simulink model "SF053A_HwAgVehCentrTrim"  (R2013b)
settings: Solver=FixedStepDiscrete  SolverMode=SingleTasking  StartTime=0.0  StopTime=1  FixedStep=0.002  RelTol=1e-3
values from neighbouring files (symbols this model uses):
  ENGRUNACTVTRUE_CNT_U08 = DataDict.Constant    [SF053A_HwAgVehCentrTrim_DataDict.m]
  HWAGCLRTRIMPRFMD_CNT_LGC = DataDict.Constant    [SF053A_HwAgVehCentrTrim_DataDict.m]
  HWAGCLRVAL_HWDEG_F32 = DataDict.Constant    [SF053A_HwAgVehCentrTrim_DataDict.m]
  HWAGEOTCCWNOTDETD_CNT_U08 = DataDict.Constant    [SF053A_HwAgVehCentrTrim_DataDict.m]
  HWAGEOTCWNOTDETD_CNT_U08 = DataDict.Constant    [SF053A_HwAgVehCentrTrim_DataDict.m]
  HWAGMAGTHDEXCDD_CNT_U08 = DataDict.Constant    [SF053A_HwAgVehCentrTrim_DataDict.m]
  HWAGTRIMPRFMD_CNT_LGC = DataDict.Constant    [SF053A_HwAgVehCentrTrim_DataDict.m]
  HwAgVehCentrTrimHwAgLim = DataDict.Calibration    [SF053A_HwAgVehCentrTrim_DataDict.m]
  HwAgVehCentrTrimVehSpdMaxThd = DataDict.Calibration    [SF053A_HwAgVehCentrTrim_DataDict.m]
  HwAgVehCentrTrimVld = DataDict.NTC    [SF053A_HwAgVehCentrTrim_DataDict.m]
  NODEBSTEP_CNT_U16 = DataDict.Constant    [SF053A_HwAgVehCentrTrim_DataDict.m]
  UPDHWAGTRIMPRFMD_CNT_U08 = DataDict.Constant    [SF053A_HwAgVehCentrTrim_DataDict.m]
  VEHSPDTHDEXCDD_CNT_U08 = DataDict.Constant    [SF053A_HwAgVehCentrTrim_DataDict.m]
undefined symbols (not defined in the file or in its folder): NtcSts1, u2, u3, u4, u5
libraries: simulink x6, NxtrNvM x3, NxtrLim x2
(part 2 of 3)

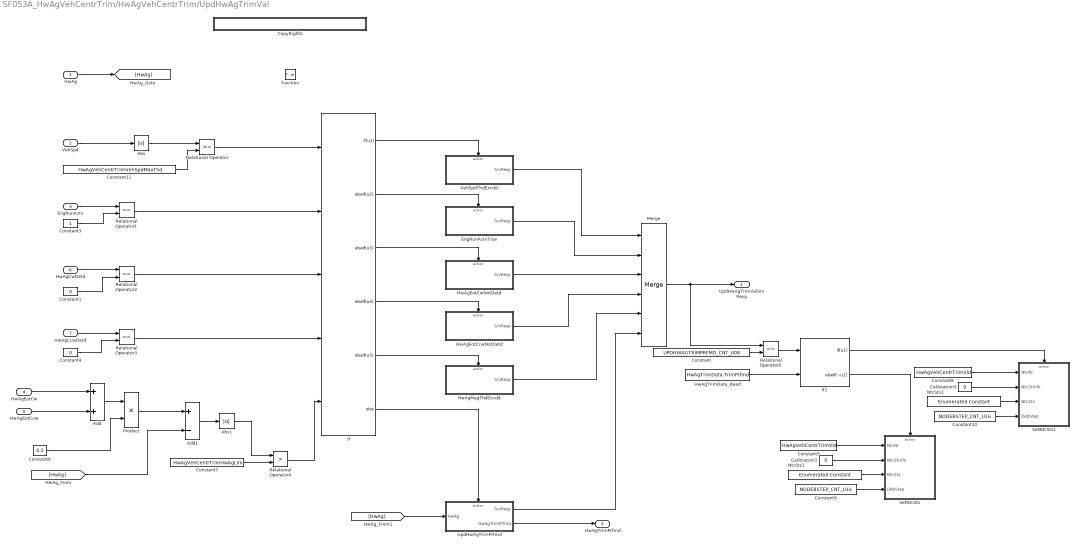
== system SF053A_HwAgVehCentrTrim/HwAgVehCentrTrim/UpdHwAgTrimVal ==
  HwAg : Inport
  VehSpd : Inport  RequirementInfo="{'linktype_rmi_doors' '0000babb (/E-STEER Core/SubSystem Specifications/Application Functions/SF053A Handwheel Angle Vehicle Center Trim)' '#SF053A_32' 'true' 'REQ:  SF053A_32' '' ; 'linktype_rmi_doors' '0000babb (/E-STEER Core/SubSystem Specifications/Application Functions/SF053A Handwheel Angle Vehicle Center Trim)' '#SF053A_79' 'true' 'REQ:  SF053A_79' '' } %GIDa_a63d72e2_7325_4356_9d1e_f8480a82d0d4"  Port=2
  EngRunActv : Inport  RequirementInfo="{'linktype_rmi_doors' '0000babb (/E-STEER Core/SubSystem Specifications/Application Functions/SF053A Handwheel Angle Vehicle Center Trim)' '#SF053A_32' 'true' 'REQ:  SF053A_32' '' ; 'linktype_rmi_doors' '0000babb (/E-STEER Core/SubSystem Specifications/Application Functions/SF053A Handwheel Angle Vehicle Center Trim)' '#SF053A_79' 'true' 'REQ:  SF053A_79' '' } %GIDa_7bfd1cfe_a81d_4c20_a64c_d0273af8ffe3"  Port=3
  HwAgEotCw : Inport  RequirementInfo="{'linktype_rmi_doors' '0000babb (/E-STEER Core/SubSystem Specifications/Application Functions/SF053A Handwheel Angle Vehicle Center Trim)' '#SF053A_32' 'true' 'REQ:  SF053A_32' '' ; 'linktype_rmi_doors' '0000babb (/E-STEER Core/SubSystem Specifications/Application Functions/SF053A Handwheel Angle Vehicle Center Trim)' '#SF053A_79' 'true' 'REQ:  SF053A_79' '' } %GIDa_18a440d3_64a6_4375_b85b_cbfdb945b10b"  Port=4
  HwAgEotCcw : Inport  RequirementInfo="{'linktype_rmi_doors' '0000babb (/E-STEER Core/SubSystem Specifications/Application Functions/SF053A Handwheel Angle Vehicle Center Trim)' '#SF053A_32' 'true' 'REQ:  SF053A_32' '' ; 'linktype_rmi_doors' '0000babb (/E-STEER Core/SubSystem Specifications/Application Functions/SF053A Handwheel Angle Vehicle Center Trim)' '#SF053A_79' 'true' 'REQ:  SF053A_79' '' } %GIDa_1e2d1dde_4459_46e8_93f9_57f17d4f6490"  Port=5
  HwAgCwDetd : Inport  RequirementInfo="{'linktype_rmi_doors' '0000babb (/E-STEER Core/SubSystem Specifications/Application Functions/SF053A Handwheel Angle Vehicle Center Trim)' '#SF053A_32' 'true' 'REQ:  SF053A_32' '' ; 'linktype_rmi_doors' '0000babb (/E-STEER Core/SubSystem Specifications/Application Functions/SF053A Handwheel Angle Vehicle Center Trim)' '#SF053A_79' 'true' 'REQ:  SF053A_79' '' } %GIDa_ce18ba93_be2d_4182_b1c9_fe28610a3b2f"  Port=6
  HwAgCcwDetd : Inport  RequirementInfo="{'linktype_rmi_doors' '0000babb (/E-STEER Core/SubSystem Specifications/Application Functions/SF053A Handwheel Angle Vehicle Center Trim)' '#SF053A_32' 'true' 'REQ:  SF053A_32' '' ; 'linktype_rmi_doors' '0000babb (/E-STEER Core/SubSystem Specifications/Application Functions/SF053A Handwheel Angle Vehicle Center Trim)' '#SF053A_79' 'true' 'REQ:  SF053A_79' '' } %GIDa_ef525b95_af54_48f7_86e9_a1604fe43558"  Port=7
  function : TriggerPort  TriggerType=function-call
  Abs : Abs  RequirementInfo="{'linktype_rmi_doors' '0000babb (/E-STEER Core/SubSystem Specifications/Application Functions/SF053A Handwheel Angle Vehicle Center Trim)' '#SF053A_32' 'true' 'REQ:  SF053A_32' '' ; 'linktype_rmi_doors' '0000babb (/E-STEER Core/SubSystem Specifications/Application Functions/SF053A Handwheel Angle Vehicle Center Trim)' '#SF053A_79' 'true' 'REQ:  SF053A_79' '' } %GIDa_d991774f_80ee_4fb7_a63e_280bffb35c40"
  Abs1 : Abs  RequirementInfo="{'linktype_rmi_doors' '0000babb (/E-STEER Core/SubSystem Specifications/Application Functions/SF053A Handwheel Angle Vehicle Center Trim)' '#SF053A_32' 'true' 'REQ:  SF053A_32' '' ; 'linktype_rmi_doors' '0000babb (/E-STEER Core/SubSystem Specifications/Application Functions/SF053A Handwheel Angle Vehicle Center Trim)' '#SF053A_79' 'true' 'REQ:  SF053A_79' '' } %GIDa_67f6e9b9_3d0b_4591_be2f_c526e2159446"
  Add : Sum  RequirementInfo="{'linktype_rmi_doors' '0000babb (/E-STEER Core/SubSystem Specifications/Application Functions/SF053A Handwheel Angle Vehicle Center Trim)' '#SF053A_32' 'true' 'REQ:  SF053A_32' '' ; 'linktype_rmi_doors' '0000babb (/E-STEER Core/SubSystem Specifications/Application Functions/SF053A Handwheel Angle Vehicle Center Trim)' '#SF053A_79' 'true' 'REQ:  SF053A_79' '' } %GIDa_2f9a8ad5_a900_41c0_be49_db9892669b9e"
  Add1 : Sum  RequirementInfo="{'linktype_rmi_doors' '0000babb (/E-STEER Core/SubSystem Specifications/Application Functions/SF053A Handwheel Angle Vehicle Center Trim)' '#SF053A_32' 'true' 'REQ:  SF053A_32' '' ; 'linktype_rmi_doors' '0000babb (/E-STEER Core/SubSystem Specifications/Application Functions/SF053A Handwheel Angle Vehicle Center Trim)' '#SF053A_79' 'true' 'REQ:  SF053A_79' '' } %GIDa_21c46d49_c724_4955_a3b5_87003d98a67a"  Inputs=+-
  Calibration1 : Constant  RequirementInfo="{'linktype_rmi_doors' '0000babb (/E-STEER Core/SubSystem Specifications/Application Functions/SF053A Handwheel Angle Vehicle Center Trim)' '#SF053A_110' 'true' 'REQ:  SF053A_110' '' } %GIDa_9f686a85_bd88_41db_9064_cadbbf5e7fb3"  Value=0  OutDataTypeStr=uint8
      settings: AttributesFormatString=%<OutDataTypeStr>
  Calibration3 : Constant  RequirementInfo="{'linktype_rmi_doors' '0000babb (/E-STEER Core/SubSystem Specifications/Application Functions/SF053A Handwheel Angle Vehicle Center Trim)' '#SF053A_111' 'true' 'REQ:  SF053A_111' '' } %GIDa_8f2b5906_6f05_4464_aae5_08c6a45211c4"  Value=0  OutDataTypeStr=uint8
      settings: AttributesFormatString=%<OutDataTypeStr>
  Constant : Constant  RequirementInfo="{'linktype_rmi_doors' '0000babb (/E-STEER Core/SubSystem Specifications/Application Functions/SF053A Handwheel Angle Vehicle Center Trim)' '#SF053A_110' 'true' 'REQ:  SF053A_110' '' ; 'linktype_rmi_doors' '0000babb (/E-STEER Core/SubSystem Specifications/Application Functions/SF053A Handwheel Angle Vehicle Center Trim)' '#SF053A_111' 'true' 'REQ:  SF053A_111' '' } %GIDa_8956af61_b54b_47ee_9afc_75d26d1ad22e"  Value=UPDHWAGTRIMPRFMD_CNT_U08
  Constant1 : Constant  RequirementInfo="{'linktype_rmi_doors' '0000babb (/E-STEER Core/SubSystem Specifications/Application Functions/SF053A Handwheel Angle Vehicle Center Trim)' '#SF053A_32' 'true' 'REQ:  SF053A_32' '' ; 'linktype_rmi_doors' '0000babb (/E-STEER Core/SubSystem Specifications/Application Functions/SF053A Handwheel Angle Vehicle Center Trim)' '#SF053A_79' 'true' 'REQ:  SF053A_79' '' } %GIDa_9589e086_47c5_4cb5_81f5_13b7ff01c35c"  Value=0
  Constant10 : Constant  RequirementInfo="{'linktype_rmi_doors' '0000babb (/E-STEER Core/SubSystem Specifications/Application Functions/SF053A Handwheel Angle Vehicle Center Trim)' '#SF053A_111' 'true' 'REQ:  SF053A_111' '' } %GIDa_c2f6ab27_85aa_4a97_8728_f108cbc9ac24"  Value=NODEBSTEP_CNT_U16
  Constant11 : Constant  RequirementInfo="{'linktype_rmi_doors' '0000babb (/E-STEER Core/SubSystem Specifications/Application Functions/SF053A Handwheel Angle Vehicle Center Trim)' '#SF053A_60' 'true' 'REQ:  SF053A_60' '' } %GIDa_d2bea2c8_1d63_41b6_a25d_09f8e76b65b2"  Value=HwAgVehCentrTrimVehSpdMaxThd
  Constant3 : Constant  RequirementInfo="{'linktype_rmi_doors' '0000babb (/E-STEER Core/SubSystem Specifications/Application Functions/SF053A Handwheel Angle Vehicle Center Trim)' '#SF053A_32' 'true' 'REQ:  SF053A_32' '' ; 'linktype_rmi_doors' '0000babb (/E-STEER Core/SubSystem Specifications/Application Functions/SF053A Handwheel Angle Vehicle Center Trim)' '#SF053A_79' 'true' 'REQ:  SF053A_79' '' } %GIDa_b075b36d_915b_4cb5_9147_9c5d0640a7d0"
  Constant4 : Constant  RequirementInfo="{'linktype_rmi_doors' '0000babb (/E-STEER Core/SubSystem Specifications/Application Functions/SF053A Handwheel Angle Vehicle Center Trim)' '#SF053A_32' 'true' 'REQ:  SF053A_32' '' ; 'linktype_rmi_doors' '0000babb (/E-STEER Core/SubSystem Specifications/Application Functions/SF053A Handwheel Angle Vehicle Center Trim)' '#SF053A_79' 'true' 'REQ:  SF053A_79' '' } %GIDa_c3d3dc4c_4260_4809_b9a5_21422385d61f"  Value=0
  Constant5 : Constant  RequirementInfo="{'linktype_rmi_doors' '0000babb (/E-STEER Core/SubSystem Specifications/Application Functions/SF053A Handwheel Angle Vehicle Center Trim)' '#SF053A_110' 'true' 'REQ:  SF053A_110' '' } %GIDa_4525d2f8_5127_471e_91b9_307fc94a9020"  Value=HwAgVehCentrTrimVld
  Constant6 : Constant  RequirementInfo="{'linktype_rmi_doors' '0000babb (/E-STEER Core/SubSystem Specifications/Application Functions/SF053A Handwheel Angle Vehicle Center Trim)' '#SF053A_32' 'true' 'REQ:  SF053A_32' '' ; 'linktype_rmi_doors' '0000babb (/E-STEER Core/SubSystem Specifications/Application Functions/SF053A Handwheel Angle Vehicle Center Trim)' '#SF053A_79' 'true' 'REQ:  SF053A_79' '' } %GIDa_69b41a62_8ab0_4c1b_8241_6f2b857f2a9c"  Value=0.5
  Constant7 : Constant  RequirementInfo="{'linktype_rmi_doors' '0000babb (/E-STEER Core/SubSystem Specifications/Application Functions/SF053A Handwheel Angle Vehicle Center Trim)' '#SF053A_32' 'true' 'REQ:  SF053A_32' '' ; 'linktype_rmi_doors' '0000babb (/E-STEER Core/SubSystem Specifications/Application Functions/SF053A Handwheel Angle Vehicle Center Trim)' '#SF053A_79' 'true' 'REQ:  SF053A_79' '' } %GIDa_c482106a_1fa7_4c73_8678_7892ee44990b"  Value=HwAgVehCentrTrimHwAgLim
  Constant8 : Constant  RequirementInfo="{'linktype_rmi_doors' '0000babb (/E-STEER Core/SubSystem Specifications/Application Functions/SF053A Handwheel Angle Vehicle Center Trim)' '#SF053A_111' 'true' 'REQ:  SF053A_111' '' } %GIDa_d51d30af_f410_42f9_8ce2_7cda550b525d"  Value=HwAgVehCentrTrimVld
  Constant9 : Constant  RequirementInfo="{'linktype_rmi_doors' '0000babb (/E-STEER Core/SubSystem Specifications/Application Functions/SF053A Handwheel Angle Vehicle Center Trim)' '#SF053A_110' 'true' 'REQ:  SF053A_110' '' } %GIDa_3258ff11_795f_4169_b902_ffcb86c32c40"  Value=NODEBSTEP_CNT_U16
  CopyRight2 : Subsystem  Description=|  mask(Copyright Information){none=on}
      | Copyright info block.                                               
      |                                                                     
      | Place copyright information at the top of every subsystem in design.
      mask prompts: none "No parameters"
      mask help: Place copyright information at the top of every subsystem in design.
      mask Display:
      | NxtrConf = 'Nexteer Confidential';
      | 
      | sys = bdroot; %handle for the current model ("system")
      | first = get_param(sys,'Created');
      | if(isempty(first))
      |     first = datestr(now,'yyyy');
      | else
      |     first = first(end-3:end);  %year is last four digits
      | end
      | 
      | last = get_param(sys,'LastModifiedDate');
      | if isempty(last)
      |     last = datestr(now,'yyyy');
      | else
      |     last = last(end-3:end);
      | end
      | 
      | if strcmp(first,last)
      |     fprintf('%s -- Copyright %s Nexteer',NxtrConf,first)
      | else
      |     fprintf('%s -- %s%s- %s Nexteer',NxtrConf,char(169),first,last)
      | end
  EngRunActvTrue : Subsystem  RequirementInfo="{'linktype_rmi_doors' '0000babb (/E-STEER Core/SubSystem Specifications/Application Functions/SF053A Handwheel Angle Vehicle Center Trim)' '#SF053A_32' 'true' 'REQ:  SF053A_32' '' ; 'linktype_rmi_doors' '0000babb (/E-STEER Core/SubSystem Specifications/Application Functions/SF053A Handwheel Angle Vehicle Center Trim)' '#SF053A_70' 'true' 'REQ:  SF053A_70' '' ; 'linktype_rmi_doors' '0000babb (/E-STEER Core/SubSystem Specifications/Application Functions/SF053A Handwheel Angle Vehicle Center Trim)' '#SF053A_72' 'true' 'REQ:  SF053A_72' '' } %GIDa_ba91543d_fb8d_4cd3_85a8_35f516007121"  TreatAsAtomicUnit=on
  HwAgEotCcwNotDetd : Subsystem  RequirementInfo="{'linktype_rmi_doors' '0000babb (/E-STEER Core/SubSystem Specifications/Application Functions/SF053A Handwheel Angle Vehicle Center Trim)' '#SF053A_32' 'true' 'REQ:  SF053A_32' '' ; 'linktype_rmi_doors' '0000babb (/E-STEER Core/SubSystem Specifications/Application Functions/SF053A Handwheel Angle Vehicle Center Trim)' '#SF053A_70' 'true' 'REQ:  SF053A_70' '' ; 'linktype_rmi_doors' '0000babb (/E-STEER Core/SubSystem Specifications/Application Functions/SF053A Handwheel Angle Vehicle Center Trim)' '#SF053A_74' 'true' 'REQ:  SF053A_74' '' } %GIDa_250d4040_571b_4921_ad24_fde6fcce09c5"  TreatAsAtomicUnit=on
  HwAgEotCwNotDetd : Subsystem  RequirementInfo="{'linktype_rmi_doors' '0000babb (/E-STEER Core/SubSystem Specifications/Application Functions/SF053A Handwheel Angle Vehicle Center Trim)' '#SF053A_32' 'true' 'REQ:  SF053A_32' '' ; 'linktype_rmi_doors' '0000babb (/E-STEER Core/SubSystem Specifications/Application Functions/SF053A Handwheel Angle Vehicle Center Trim)' '#SF053A_70' 'true' 'REQ:  SF053A_70' '' ; 'linktype_rmi_doors' '0000babb (/E-STEER Core/SubSystem Specifications/Application Functions/SF053A Handwheel Angle Vehicle Center Trim)' '#SF053A_73' 'true' 'REQ:  SF053A_73' '' } %GIDa_52a5771d_f986_44c5_b47b_cdbc55140e93"  TreatAsAtomicUnit=on
  HwAgMagThdExcdd : Subsystem  RequirementInfo="{'linktype_rmi_doors' '0000babb (/E-STEER Core/SubSystem Specifications/Application Functions/SF053A Handwheel Angle Vehicle Center Trim)' '#SF053A_32' 'true' 'REQ:  SF053A_32' '' ; 'linktype_rmi_doors' '0000babb (/E-STEER Core/SubSystem Specifications/Application Functions/SF053A Handwheel Angle Vehicle Center Trim)' '#SF053A_70' 'true' 'REQ:  SF053A_70' '' ; 'linktype_rmi_doors' '0000babb (/E-STEER Core/SubSystem Specifications/Application Functions/SF053A Handwheel Angle Vehicle Center Trim)' '#SF053A_75' 'true' 'REQ:  SF053A_75' '' } %GIDa_589bbf88_c4ec_407b_bfba_557710da451a"  TreatAsAtomicUnit=on
  HwAgTrimData_Read : DataStoreRead  RequirementInfo="{'linktype_rmi_doors' '0000babb (/E-STEER Core/SubSystem Specifications/Application Functions/SF053A Handwheel Angle Vehicle Center Trim)' '#SF053A_110' 'true' 'REQ:  SF053A_110' '' ; 'linktype_rmi_doors' '0000babb (/E-STEER Core/SubSystem Specifications/Application Functions/SF053A Handwheel Angle Vehicle Center Trim)' '#SF053A_111' 'true' 'REQ:  SF053A_111' '' } %GIDa_1228ea93_d8e8_46bc_b526_ed5b914aa260"  DataStoreName=HwAgTrimData  DataStoreElements=HwAgTrimData.TrimPrfmd
  If : If  RequirementInfo="{'linktype_rmi_doors' '0000babb (/E-STEER Core/SubSystem Specifications/Application Functions/SF053A Handwheel Angle Vehicle Center Trim)' '#SF053A_32' 'true' 'REQ:  SF053A_32' '' } %GIDa_2a546bba_ef04_4de4_a412_fac081507659"  NumInputs=5  IfExpression=u1  ElseIfExpressions=u2,u3,u4,u5
  If1 : If  RequirementInfo="{'linktype_rmi_doors' '0000babb (/E-STEER Core/SubSystem Specifications/Application Functions/SF053A Handwheel Angle Vehicle Center Trim)' '#SF053A_110' 'true' 'REQ:  SF053A_110' '' ; 'linktype_rmi_doors' '0000babb (/E-STEER Core/SubSystem Specifications/Application Functions/SF053A Handwheel Angle Vehicle Center Trim)' '#SF053A_111' 'true' 'REQ:  SF053A_111' '' } %GIDa_f78b1e01_142e_43af_ba95_66698126f979"  NumInputs=2  IfExpression=u1  ElseIfExpressions=~u2  ShowElse=off
  Merge : Merge  RequirementInfo="{'linktype_rmi_doors' '0000babb (/E-STEER Core/SubSystem Specifications/Application Functions/SF053A Handwheel Angle Vehicle Center Trim)' '#SF053A_32' 'true' 'REQ:  SF053A_32' '' } %GIDa_df60f44e_6141_4196_a81c_516d305baf5c"  Inputs=6
  NtcSts1 : simulink/Sources/Enumerated Constant  RequirementInfo="{'linktype_rmi_doors' '0000babb (/E-STEER Core/SubSystem Specifications/Application Functions/SF053A Handwheel Angle Vehicle Center Trim)' '#SF053A_110' 'true' 'REQ:  SF053A_110' '' } %GIDa_8192f31f_0ad0_4e20_8a98_bf7e939c383f"  OutDataTypeStr=Enum: NtcSts1  Value=NtcSts1.NTCSTS_FAILD  SampleTime=inf
  NtcSts2 : simulink/Sources/Enumerated Constant  RequirementInfo="{'linktype_rmi_doors' '0000babb (/E-STEER Core/SubSystem Specifications/Application Functions/SF053A Handwheel Angle Vehicle Center Trim)' '#SF053A_111' 'true' 'REQ:  SF053A_111' '' } %GIDa_0b84bfc1_5cc9_49c6_9963_bea2df097407"  OutDataTypeStr=Enum: NtcSts1  Value=NtcSts1.NTCSTS_PASSD  SampleTime=inf
  Product : Product  RequirementInfo="{'linktype_rmi_doors' '0000babb (/E-STEER Core/SubSystem Specifications/Application Functions/SF053A Handwheel Angle Vehicle Center Trim)' '#SF053A_32' 'true' 'REQ:  SF053A_32' '' ; 'linktype_rmi_doors' '0000babb (/E-STEER Core/SubSystem Specifications/Application Functions/SF053A Handwheel Angle Vehicle Center Trim)' '#SF053A_79' 'true' 'REQ:  SF053A_79' '' } %GIDa_91f1eb26_be4f_4e76_a9d8_c63b551ee0fb"
  Relational Operator : RelationalOperator  RequirementInfo="{'linktype_rmi_doors' '0000babb (/E-STEER Core/SubSystem Specifications/Application Functions/SF053A Handwheel Angle Vehicle Center Trim)' '#SF053A_32' 'true' 'REQ:  SF053A_32' '' ; 'linktype_rmi_doors' '0000babb (/E-STEER Core/SubSystem Specifications/Application Functions/SF053A Handwheel Angle Vehicle Center Trim)' '#SF053A_79' 'true' 'REQ:  SF053A_79' '' } %GIDa_3c5aa961_edb7_4924_8f97_d3c54525646e"  OutDataTypeStr=boolean
  Relational Operator1 : RelationalOperator  RequirementInfo="{'linktype_rmi_doors' '0000babb (/E-STEER Core/SubSystem Specifications/Application Functions/SF053A Handwheel Angle Vehicle Center Trim)' '#SF053A_32' 'true' 'REQ:  SF053A_32' '' ; 'linktype_rmi_doors' '0000babb (/E-STEER Core/SubSystem Specifications/Application Functions/SF053A Handwheel Angle Vehicle Center Trim)' '#SF053A_79' 'true' 'REQ:  SF053A_79' '' } %GIDa_637e2b68_db5e_4c81_9032_9ca0fccded3e"  Operator===  OutDataTypeStr=boolean
  Relational Operator2 : RelationalOperator  RequirementInfo="{'linktype_rmi_doors' '0000babb (/E-STEER Core/SubSystem Specifications/Application Functions/SF053A Handwheel Angle Vehicle Center Trim)' '#SF053A_32' 'true' 'REQ:  SF053A_32' '' ; 'linktype_rmi_doors' '0000babb (/E-STEER Core/SubSystem Specifications/Application Functions/SF053A Handwheel Angle Vehicle Center Trim)' '#SF053A_79' 'true' 'REQ:  SF053A_79' '' } %GIDa_54ad7389_ac17_4e5b_a3db_98a413908bf6"  Operator===  OutDataTypeStr=boolean
  Relational Operator3 : RelationalOperator  RequirementInfo="{'linktype_rmi_doors' '0000babb (/E-STEER Core/SubSystem Specifications/Application Functions/SF053A Handwheel Angle Vehicle Center Trim)' '#SF053A_32' 'true' 'REQ:  SF053A_32' '' ; 'linktype_rmi_doors' '0000babb (/E-STEER Core/SubSystem Specifications/Application Functions/SF053A Handwheel Angle Vehicle Center Trim)' '#SF053A_79' 'true' 'REQ:  SF053A_79' '' } %GIDa_4fb7c085_ee2d_4650_a5d6_c2cd77fefe3e"  Operator===  OutDataTypeStr=boolean
  Relational Operator4 : RelationalOperator  RequirementInfo="{'linktype_rmi_doors' '0000babb (/E-STEER Core/SubSystem Specifications/Application Functions/SF053A Handwheel Angle Vehicle Center Trim)' '#SF053A_32' 'true' 'REQ:  SF053A_32' '' ; 'linktype_rmi_doors' '0000babb (/E-STEER Core/SubSystem Specifications/Application Functions/SF053A Handwheel Angle Vehicle Center Trim)' '#SF053A_79' 'true' 'REQ:  SF053A_79' '' } %GIDa_d472fc75_b451_4178_9f76_6ec74d7051b5"  Operator=>  OutDataTypeStr=boolean
  Relational Operator5 : RelationalOperator  RequirementInfo="{'linktype_rmi_doors' '0000babb (/E-STEER Core/SubSystem Specifications/Application Functions/SF053A Handwheel Angle Vehicle Center Trim)' '#SF053A_110' 'true' 'REQ:  SF053A_110' '' ; 'linktype_rmi_doors' '0000babb (/E-STEER Core/SubSystem Specifications/Application Functions/SF053A Handwheel Angle Vehicle Center Trim)' '#SF053A_111' 'true' 'REQ:  SF053A_111' '' } %GIDa_9ea5f935_7222_4a4e_bd22_5588c83f4498"  Operator===  OutDataTypeStr=boolean
  SetNtcSts : Subsystem  RequirementInfo="{'linktype_rmi_doors' '0000babb (/E-STEER Core/SubSystem Specifications/Application Functions/SF053A Handwheel Angle Vehicle Center Trim)' '#SF053A_110' 'true' 'REQ:  SF053A_110' '' } %GIDa_4621e7e0_cc57_4ab8_9e39_f2c96da631c5"  mask(SetNTC){}
      mask help: SetNTC library block
  SetNtcSts1 : Subsystem  RequirementInfo="{'linktype_rmi_doors' '0000babb (/E-STEER Core/SubSystem Specifications/Application Functions/SF053A Handwheel Angle Vehicle Center Trim)' '#SF053A_111' 'true' 'REQ:  SF053A_111' '' } %GIDa_653df0eb_523c_4973_ade4_5ccb12e6fe5a"  mask(SetNTC){}
      mask help: SetNTC library block
  UpdHwAgTrimPrfmd : Subsystem  TreatAsAtomicUnit=on
  VehSpdThdExcdd : Subsystem  RequirementInfo="{'linktype_rmi_doors' '0000babb (/E-STEER Core/SubSystem Specifications/Application Functions/SF053A Handwheel Angle Vehicle Center Trim)' '#SF053A_32' 'true' 'REQ:  SF053A_32' '' ; 'linktype_rmi_doors' '0000babb (/E-STEER Core/SubSystem Specifications/Application Functions/SF053A Handwheel Angle Vehicle Center Trim)' '#SF053A_70' 'true' 'REQ:  SF053A_70' '' ; 'linktype_rmi_doors' '0000babb (/E-STEER Core/SubSystem Specifications/Application Functions/SF053A Handwheel Angle Vehicle Center Trim)' '#SF053A_71' 'true' 'REQ:  SF053A_71' '' } %GIDa_cf061c3e_81c2_4250_a488_ce9352259aa5"  TreatAsAtomicUnit=on
  UpdHwAgTrimValSrvResp : Outport  RequirementInfo="{'linktype_rmi_doors' '0000babb (/E-STEER Core/SubSystem Specifications/Application Functions/SF053A Handwheel Angle Vehicle Center Trim)' '#SF053A_32' 'true' 'REQ:  SF053A_32' '' } %GIDa_585df83e_3fcf_4b36_b22c_e3be5ff7056c"
  HwAgTrimPrfmd : Outport  Port=2
  wires:
  Constant8/1 -> SetNtcSts1/1(NtcNr)
  Constant5/1 -> SetNtcSts/1(NtcNr)
  VehSpd/1 -> Abs/1
  Abs/1 -> Relational Operator/1
  Constant11/1 -> Relational Operator/2
  EngRunActv/1 -> Relational Operator1/1
  Constant3/1 -> Relational Operator1/2
  HwAgCwDetd/1 -> Relational Operator2/1
  Constant1/1 -> Relational Operator2/2
  HwAgCcwDetd/1 -> Relational Operator3/1
  Constant4/1 -> Relational Operator3/2
  Add/1 -> Product/1
  Constant6/1 -> Product/2
  Product/1 -> Add1/1
  [HwAg] -> Add1/2
  Add1/1 -> Abs1/1
  Constant7/1 -> Relational Operator4/2
  Relational Operator4/1 -> If/5
  Relational Operator/1 -> If/1
  Relational Operator1/1 -> If/2
  Relational Operator2/1 -> If/3
  Relational Operator3/1 -> If/4
  HwAg/1 -> [HwAg]
  If/1 -> VehSpdThdExcdd/Action
  If/2 -> EngRunActvTrue/Action
  If/3 -> HwAgEotCwNotDetd/Action
  If/4 -> HwAgEotCcwNotDetd/Action
  If/5 -> HwAgMagThdExcdd/Action
  If/6 -> UpdHwAgTrimPrfmd/Action
  HwAgEotCcwNotDetd/1(SrvResp) -> Merge/4
  HwAgEotCwNotDetd/1(SrvResp) -> Merge/3
  HwAgMagThdExcdd/1(SrvResp) -> Merge/5
  EngRunActvTrue/1(SrvResp) -> Merge/2
  UpdHwAgTrimPrfmd/1(SrvResp) -> Merge/6
  VehSpdThdExcdd/1(SrvResp) -> Merge/1
  Merge/1 -> Relational Operator5/1, UpdHwAgTrimValSrvResp/1
  [HwAg] -> UpdHwAgTrimPrfmd/1(HwAg)
  Abs1/1 -> Relational Operator4/1
  HwAgEotCw/1 -> Add/1
  HwAgEotCcw/1 -> Add/2
  UpdHwAgTrimPrfmd/2(HwAgTrimPrfmd) -> HwAgTrimPrfmd/1
  NtcSts1/1 -> SetNtcSts/3(NtcSts)
  Constant9/1 -> SetNtcSts/4(DebStep)
  Calibration1/1 -> SetNtcSts/2(NtcStInfo)
  Relational Operator5/1 -> If1/1
  Constant/1 -> Relational Operator5/2
  If1/2 -> SetNtcSts/Action
  NtcSts2/1 -> SetNtcSts1/3(NtcSts)
  Constant10/1 -> SetNtcSts1/4(DebStep)
  Calibration3/1 -> SetNtcSts1/2(NtcStInfo)
  If1/1 -> SetNtcSts1/Action
  HwAgTrimData_Read/1 -> If1/2

== system SF053A_HwAgVehCentrTrim/HwAgVehCentrTrim/ClrHwAgTrimVal/CopyRight2 ==

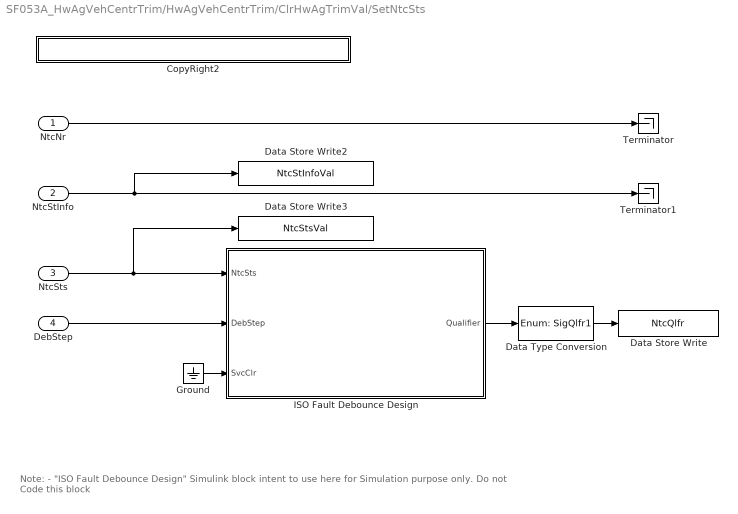
== system SF053A_HwAgVehCentrTrim/HwAgVehCentrTrim/ClrHwAgTrimVal/SetNtcSts ==
  note: Note:
      |
      | - "ISO Fault Debounce Design" Simulink block intent to use here for Simulation purpose only. Do not Code this block
  NtcNr : Inport
  NtcStInfo : Inport  Port=2
  NtcSts : Inport  Port=3
  DebStep : Inport  Port=4
  CopyRight2 : Subsystem  Description=|  mask(Copyright Information){none=on}
      | Copyright info block.                                               
      |                                                                     
      | Place copyright information at the top of every subsystem in design.
      mask prompts: none "No parameters"
      mask help: Place copyright information at the top of every subsystem in design.
      mask Display:
      | NxtrConf = 'Nexteer Confidential';
      | 
      | sys = bdroot; %handle for the current model ("system")
      | first = get_param(sys,'Created');
      | first = first(end-3:end);  %year is last four digits
      | 
      | last = get_param(sys,'LastModifiedDate');
      | if isempty(last)
      |     last = datestr(now,'yyyy');
      | else
      |     last = last(end-3:end);
      | end
      | 
      | if strcmp(first,last)
      |     fprintf('%s -- Copyright %s Nexteer',NxtrConf,first)
      | else
      |     fprintf('%s -- %s%s- %s Nexteer',NxtrConf,char(169),first,last)
      | end
  Data Store Write : DataStoreWrite  DataStoreName=NtcQlfr
  Data Store Write2 : DataStoreWrite  DataStoreName=NtcStInfoVal
  Data Store Write3 : DataStoreWrite  DataStoreName=NtcStsVal
  Data Type Conversion : DataTypeConversion  OutDataTypeStr=Enum: SigQlfr1
  Ground : Ground
  ISO Fault Debounce Design : Stateflow chart  TreatAsAtomicUnit=on
      settings: AttributesFormatString=|
      | Simulation Purpose Only.
      | Do Not Code this block
      | Diagnostic Manager Owns this requirement
  Terminator : Terminator
  Terminator1 : Terminator
  wires:
  NtcStInfo/1 -> Data Store Write2/1, Terminator1/1
  NtcNr/1 -> Terminator/1
  NtcSts/1 -> Data Store Write3/1, ISO Fault Debounce Design/1(NtcSts)
  DebStep/1 -> ISO Fault Debounce Design/2(DebStep)
  ISO Fault Debounce Design/1(Qualifier) -> Data Type Conversion/1
  Ground/1 -> ISO Fault Debounce Design/3(SvcClr)
  Data Type Conversion/1 -> Data Store Write/1

== system SF053A_HwAgVehCentrTrim/HwAgVehCentrTrim/GetHwAgTrimVal/CopyRight2 ==

== system SF053A_HwAgVehCentrTrim/HwAgVehCentrTrim/HwAgVehCentrTrimInit1/CopyRight2 ==

== system SF053A_HwAgVehCentrTrim/HwAgVehCentrTrim/HwAgVehCentrTrimInit1/SetNtcSts ==
  NtcNr : Inport
  NtcStInfo : Inport  Port=2
  NtcSts : Inport  Port=3
  DebStep : Inport  Port=4
  CallDiagMgr : ActionPort  ActionType=then
  CopyRight2 : Subsystem  Description=|  mask(Copyright Information){none=on}
      | Copyright info block.                                               
      |                                                                     
      | Place copyright information at the top of every subsystem in design.
      mask prompts: none "No parameters"
      mask help: Place copyright information at the top of every subsystem in design.
      mask Display:
      | NxtrConf = 'Nexteer Confidential';
      | 
      | sys = bdroot; %handle for the current model ("system")
      | first = get_param(sys,'Created');
      | if(isempty(first))
      |     first = datestr(now,'yyyy');
      | else
      |     first = first(end-3:end);  %year is last four digits
      | end
      | 
      | last = get_param(sys,'LastModifiedDate');
      | if isempty(last)
      |     last = datestr(now,'yyyy');
      | else
      |     last = last(end-3:end);
      | end
      | 
      | if strcmp(first,last)
      |     fprintf('%s -- Copyright %s Nexteer',NxtrConf,first)
      | else
      |     fprintf('%s -- %s%s- %s Nexteer',NxtrConf,char(169),first,last)
      | end
  SetNtcSts : Subsystem  RequirementInfo={} %GIDa_f65a5803_728a_455f_8230_774e70a0bec9  TreatAsAtomicUnit=on
      settings: RTWSystemCode=Inline
  wires:
  NtcNr/1 -> SetNtcSts/1(NtcNr)  "NtcNr"
  NtcSts/1 -> SetNtcSts/3(NtcSts)
  DebStep/1 -> SetNtcSts/4(DebStep)
  NtcStInfo/1 -> SetNtcSts/2(NtcStInfo)

== system SF053A_HwAgVehCentrTrim/HwAgVehCentrTrim/HwAgVehCentrTrimPer1/CopyRight2 ==

== system SF053A_HwAgVehCentrTrim/HwAgVehCentrTrim/HwAgVehCentrTrimPer1/SetNtcSts ==
  NtcNr : Inport
  NtcStInfo : Inport  Port=2
  NtcSts : Inport  Port=3
  DebStep : Inport  Port=4
  CallDiagMgr : ActionPort  ActionType=then
  CopyRight2 : Subsystem  Description=|  mask(Copyright Information){none=on}
      | Copyright info block.                                               
      |                                                                     
      | Place copyright information at the top of every subsystem in design.
      mask prompts: none "No parameters"
      mask help: Place copyright information at the top of every subsystem in design.
      mask Display:
      | NxtrConf = 'Nexteer Confidential';
      | 
      | sys = bdroot; %handle for the current model ("system")
      | first = get_param(sys,'Created');
      | if(isempty(first))
      |     first = datestr(now,'yyyy');
      | else
      |     first = first(end-3:end);  %year is last four digits
      | end
      | 
      | last = get_param(sys,'LastModifiedDate');
      | if isempty(last)
      |     last = datestr(now,'yyyy');
      | else
      |     last = last(end-3:end);
      | end
      | 
      | if strcmp(first,last)
      |     fprintf('%s -- Copyright %s Nexteer',NxtrConf,first)
      | else
      |     fprintf('%s -- %s%s- %s Nexteer',NxtrConf,char(169),first,last)
      | end
  SetNtcSts : Subsystem  RequirementInfo={} %GIDa_46a2b718_8e70_4ffb_b2e5_654f31f2fb34  TreatAsAtomicUnit=on
      settings: RTWSystemCode=Inline
  wires:
  NtcNr/1 -> SetNtcSts/1(NtcNr)  "NtcNr"
  NtcSts/1 -> SetNtcSts/3(NtcSts)
  DebStep/1 -> SetNtcSts/4(DebStep)
  NtcStInfo/1 -> SetNtcSts/2(NtcStInfo)

== system SF053A_HwAgVehCentrTrim/HwAgVehCentrTrim/SetHwAgTrimVal/CopyRight2 ==

== system SF053A_HwAgVehCentrTrim/HwAgVehCentrTrim/UpdHwAgTrimVal/CopyRight2 ==

== system SF053A_HwAgVehCentrTrim/HwAgVehCentrTrim/UpdHwAgTrimVal/EngRunActvTrue ==
  Action Port : ActionPort  ActionType=elseif
  Constant : Constant  Value=ENGRUNACTVTRUE_CNT_U08
  CopyRight2 : Subsystem  Description=|  mask(Copyright Information){none=on}
      | Copyright info block.                                               
      |                                                                     
      | Place copyright information at the top of every subsystem in design.
      mask prompts: none "No parameters"
      mask help: Place copyright information at the top of every subsystem in design.
      mask Display:
      | NxtrConf = 'Nexteer Confidential';
      | 
      | sys = bdroot; %handle for the current model ("system")
      | first = get_param(sys,'Created');
      | if(isempty(first))
      |     first = datestr(now,'yyyy');
      | else
      |     first = first(end-3:end);  %year is last four digits
      | end
      | 
      | last = get_param(sys,'LastModifiedDate');
      | if isempty(last)
      |     last = datestr(now,'yyyy');
      | else
      |     last = last(end-3:end);
      | end
      | 
      | if strcmp(first,last)
      |     fprintf('%s -- Copyright %s Nexteer',NxtrConf,first)
      | else
      |     fprintf('%s -- %s%s- %s Nexteer',NxtrConf,char(169),first,last)
      | end
  SrvResp : Outport
  wires:
  Constant/1 -> SrvResp/1

== system SF053A_HwAgVehCentrTrim/HwAgVehCentrTrim/UpdHwAgTrimVal/HwAgEotCcwNotDetd ==
  Action Port : ActionPort  ActionType=elseif
  Constant : Constant  Value=HWAGEOTCCWNOTDETD_CNT_U08
  CopyRight2 : Subsystem  Description=|  mask(Copyright Information){none=on}
      | Copyright info block.                                               
      |                                                                     
      | Place copyright information at the top of every subsystem in design.
      mask prompts: none "No parameters"
      mask help: Place copyright information at the top of every subsystem in design.
      mask Display:
      | NxtrConf = 'Nexteer Confidential';
      | 
      | sys = bdroot; %handle for the current model ("system")
      | first = get_param(sys,'Created');
      | if(isempty(first))
      |     first = datestr(now,'yyyy');
      | else
      |     first = first(end-3:end);  %year is last four digits
      | end
      | 
      | last = get_param(sys,'LastModifiedDate');
      | if isempty(last)
      |     last = datestr(now,'yyyy');
      | else
      |     last = last(end-3:end);
      | end
      | 
      | if strcmp(first,last)
      |     fprintf('%s -- Copyright %s Nexteer',NxtrConf,first)
      | else
      |     fprintf('%s -- %s%s- %s Nexteer',NxtrConf,char(169),first,last)
      | end
  SrvResp : Outport
  wires:
  Constant/1 -> SrvResp/1

== system SF053A_HwAgVehCentrTrim/HwAgVehCentrTrim/UpdHwAgTrimVal/HwAgEotCwNotDetd ==
  Action Port : ActionPort  ActionType=elseif
  Constant : Constant  Value=HWAGEOTCWNOTDETD_CNT_U08
  CopyRight2 : Subsystem  Description=|  mask(Copyright Information){none=on}
      | Copyright info block.                                               
      |                                                                     
      | Place copyright information at the top of every subsystem in design.
      mask prompts: none "No parameters"
      mask help: Place copyright information at the top of every subsystem in design.
      mask Display:
      | NxtrConf = 'Nexteer Confidential';
      | 
      | sys = bdroot; %handle for the current model ("system")
      | first = get_param(sys,'Created');
      | if(isempty(first))
      |     first = datestr(now,'yyyy');
      | else
      |     first = first(end-3:end);  %year is last four digits
      | end
      | 
      | last = get_param(sys,'LastModifiedDate');
      | if isempty(last)
      |     last = datestr(now,'yyyy');
      | else
      |     last = last(end-3:end);
      | end
      | 
      | if strcmp(first,last)
      |     fprintf('%s -- Copyright %s Nexteer',NxtrConf,first)
      | else
      |     fprintf('%s -- %s%s- %s Nexteer',NxtrConf,char(169),first,last)
      | end
  SrvResp : Outport
  wires:
  Constant/1 -> SrvResp/1

== system SF053A_HwAgVehCentrTrim/HwAgVehCentrTrim/UpdHwAgTrimVal/HwAgMagThdExcdd ==
  Action Port : ActionPort  ActionType=elseif
  Constant : Constant  Value=HWAGMAGTHDEXCDD_CNT_U08
  CopyRight2 : Subsystem  Description=|  mask(Copyright Information){none=on}
      | Copyright info block.                                               
      |                                                                     
      | Place copyright information at the top of every subsystem in design.
      mask prompts: none "No parameters"
      mask help: Place copyright information at the top of every subsystem in design.
      mask Display:
      | NxtrConf = 'Nexteer Confidential';
      | 
      | sys = bdroot; %handle for the current model ("system")
      | first = get_param(sys,'Created');
      | if(isempty(first))
      |     first = datestr(now,'yyyy');
      | else
      |     first = first(end-3:end);  %year is last four digits
      | end
      | 
      | last = get_param(sys,'LastModifiedDate');
      | if isempty(last)
      |     last = datestr(now,'yyyy');
      | else
      |     last = last(end-3:end);
      | end
      | 
      | if strcmp(first,last)
      |     fprintf('%s -- Copyright %s Nexteer',NxtrConf,first)
      | else
      |     fprintf('%s -- %s%s- %s Nexteer',NxtrConf,char(169),first,last)
      | end
  SrvResp : Outport
  wires:
  Constant/1 -> SrvResp/1

== system SF053A_HwAgVehCentrTrim/HwAgVehCentrTrim/UpdHwAgTrimVal/SetNtcSts ==
  NtcNr : Inport
  NtcStInfo : Inport  Port=2
  NtcSts : Inport  Port=3
  DebStep : Inport  Port=4
  CallDiagMgr : ActionPort  ActionType=elseif
  CopyRight2 : Subsystem  Description=|  mask(Copyright Information){none=on}
      | Copyright info block.                                               
      |                                                                     
      | Place copyright information at the top of every subsystem in design.
      mask prompts: none "No parameters"
      mask help: Place copyright information at the top of every subsystem in design.
      mask Display:
      | NxtrConf = 'Nexteer Confidential';
      | 
      | sys = bdroot; %handle for the current model ("system")
      | first = get_param(sys,'Created');
      | if(isempty(first))
      |     first = datestr(now,'yyyy');
      | else
      |     first = first(end-3:end);  %year is last four digits
      | end
      | 
      | last = get_param(sys,'LastModifiedDate');
      | if isempty(last)
      |     last = datestr(now,'yyyy');
      | else
      |     last = last(end-3:end);
      | end
      | 
      | if strcmp(first,last)
      |     fprintf('%s -- Copyright %s Nexteer',NxtrConf,first)
      | else
      |     fprintf('%s -- %s%s- %s Nexteer',NxtrConf,char(169),first,last)
      | end
  SetNtcSts : Subsystem  RequirementInfo={} %GIDa_8ac8a5ac_6b28_4b13_bed5_df7a4ec63f50  TreatAsAtomicUnit=on
      settings: RTWSystemCode=Inline
  wires:
  NtcNr/1 -> SetNtcSts/1(NtcNr)  "NtcNr"
  NtcSts/1 -> SetNtcSts/3(NtcSts)
  DebStep/1 -> SetNtcSts/4(DebStep)
  NtcStInfo/1 -> SetNtcSts/2(NtcStInfo)

== system SF053A_HwAgVehCentrTrim/HwAgVehCentrTrim/UpdHwAgTrimVal/SetNtcSts1 ==
  NtcNr : Inport
  NtcStInfo : Inport  Port=2
  NtcSts : Inport  Port=3
  DebStep : Inport  Port=4
  CallDiagMgr : ActionPort  ActionType=then
  CopyRight2 : Subsystem  Description=|  mask(Copyright Information){none=on}
      | Copyright info block.                                               
      |                                                                     
      | Place copyright information at the top of every subsystem in design.
      mask prompts: none "No parameters"
      mask help: Place copyright information at the top of every subsystem in design.
      mask Display:
      | NxtrConf = 'Nexteer Confidential';
      | 
      | sys = bdroot; %handle for the current model ("system")
      | first = get_param(sys,'Created');
      | if(isempty(first))
      |     first = datestr(now,'yyyy');
      | else
      |     first = first(end-3:end);  %year is last four digits
      | end
      | 
      | last = get_param(sys,'LastModifiedDate');
      | if isempty(last)
      |     last = datestr(now,'yyyy');
      | else
      |     last = last(end-3:end);
      | end
      | 
      | if strcmp(first,last)
      |     fprintf('%s -- Copyright %s Nexteer',NxtrConf,first)
      | else
      |     fprintf('%s -- %s%s- %s Nexteer',NxtrConf,char(169),first,last)
      | end
  SetNtcSts : Subsystem  RequirementInfo={} %GIDa_1daa32ff_5af5_4f53_9c99_9dd7ac8d1be1  TreatAsAtomicUnit=on
      settings: RTWSystemCode=Inline
  wires:
  NtcNr/1 -> SetNtcSts/1(NtcNr)  "NtcNr"
  NtcSts/1 -> SetNtcSts/3(NtcSts)
  DebStep/1 -> SetNtcSts/4(DebStep)
  NtcStInfo/1 -> SetNtcSts/2(NtcStInfo)

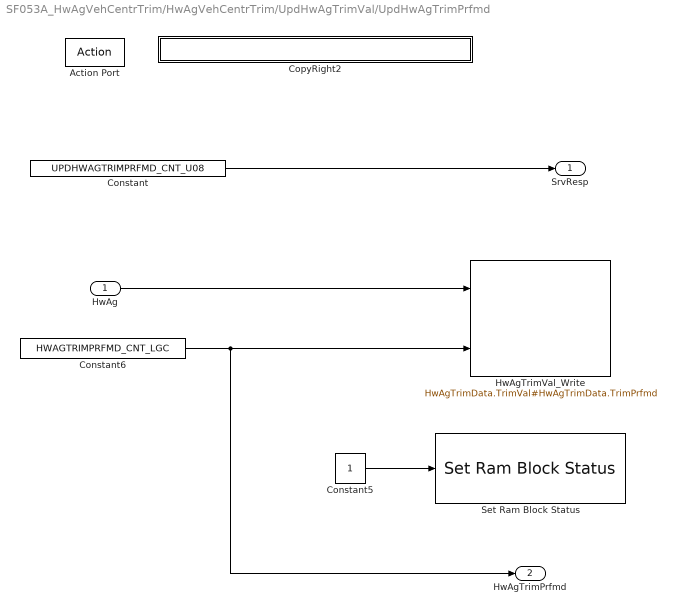
== system SF053A_HwAgVehCentrTrim/HwAgVehCentrTrim/UpdHwAgTrimVal/UpdHwAgTrimPrfmd ==
  HwAg : Inport
  Action Port : ActionPort  ActionType=else
  Constant : Constant  RequirementInfo="{'linktype_rmi_doors' '0000babb (/E-STEER Core/SubSystem Specifications/Application Functions/SF053A Handwheel Angle Vehicle Center Trim)' '#SF053A_28' 'true' 'REQ:  SF053A_28' '' } %GIDa_1c5b29d5_de90_4afe_af37_833d8f2e5eb9"  Value=UPDHWAGTRIMPRFMD_CNT_U08
  Constant5 : Constant  RequirementInfo="{'linktype_rmi_doors' '0000babb (/E-STEER Core/SubSystem Specifications/Application Functions/SF053A Handwheel Angle Vehicle Center Trim)' '#SF053A_88' 'true' 'REQ:  SF053A_88' '' ; 'linktype_rmi_doors' '0000babb (/E-STEER Core/SubSystem Specifications/Application Functions/SF053A Handwheel Angle Vehicle Center Trim)' '#SF053A_91' 'true' 'REQ:  SF053A_91' '' } %GIDa_9ca0b1c8_1b40_41ad_91d9_9a34292e68ff"  OutDataTypeStr=uint8
  Constant6 : Constant  RequirementInfo="{'linktype_rmi_doors' '0000babb (/E-STEER Core/SubSystem Specifications/Application Functions/SF053A Handwheel Angle Vehicle Center Trim)' '#SF053A_88' 'true' 'REQ:  SF053A_88' '' ; 'linktype_rmi_doors' '0000babb (/E-STEER Core/SubSystem Specifications/Application Functions/SF053A Handwheel Angle Vehicle Center Trim)' '#SF053A_91' 'true' 'REQ:  SF053A_91' '' } %GIDa_8b5d5411_3c16_41bb_9348_a58033af73af"  Value=HWAGTRIMPRFMD_CNT_LGC
  CopyRight2 : Subsystem  Description=|  mask(Copyright Information){none=on}
      | Copyright info block.                                               
      |                                                                     
      | Place copyright information at the top of every subsystem in design.
      mask prompts: none "No parameters"
      mask help: Place copyright information at the top of every subsystem in design.
      mask Display:
      | NxtrConf = 'Nexteer Confidential';
      | 
      | sys = bdroot; %handle for the current model ("system")
      | first = get_param(sys,'Created');
      | if(isempty(first))
      |     first = datestr(now,'yyyy');
      | else
      |     first = first(end-3:end);  %year is last four digits
      | end
      | 
      | last = get_param(sys,'LastModifiedDate');
      | if isempty(last)
      |     last = datestr(now,'yyyy');
      | else
      |     last = last(end-3:end);
      | end
      | 
      | if strcmp(first,last)
      |     fprintf('%s -- Copyright %s Nexteer',NxtrConf,first)
      | else
      |     fprintf('%s -- %s%s- %s Nexteer',NxtrConf,char(169),first,last)
      | end
  HwAgTrimVal_Write : DataStoreWrite  RequirementInfo="{'linktype_rmi_doors' '0000babb (/E-STEER Core/SubSystem Specifications/Application Functions/SF053A Handwheel Angle Vehicle Center Trim)' '#SF053A_88' 'true' 'REQ:  SF053A_88' '' ; 'linktype_rmi_doors' '0000babb (/E-STEER Core/SubSystem Specifications/Application Functions/SF053A Handwheel Angle Vehicle Center Trim)' '#SF053A_91' 'true' 'REQ:  SF053A_91' '' } %GIDa_76d75f5b_6889_426f_a810_cd99bb0b4047"  DataStoreName=HwAgTrimData  DataStoreElements=HwAgTrimData.TrimVal#HwAgTrimData.TrimPrfmd
  Set Ram Block Status : NxtrNvM/Set Ram Block Status  RequirementInfo="{'linktype_rmi_doors' '0000babb (/E-STEER Core/SubSystem Specifications/Application Functions/SF053A Handwheel Angle Vehicle Center Trim)' '#SF053A_88' 'true' 'REQ:  SF053A_88' '' ; 'linktype_rmi_doors' '0000babb (/E-STEER Core/SubSystem Specifications/Application Functions/SF053A Handwheel Angle Vehicle Center Trim)' '#SF053A_91' 'true' 'REQ:  SF053A_91' '' } %GIDa_f63863d1_de55_46b8_b756_de4e9a486ee5"  FuncName=Set Ram Block Status  NvMBlockName=HwAgTrimData  VoidFuncRtn=on  BlockChanged_DSN=NvMSRBS_BlockChanged  Return_DSN=NvMSRBS_Return
      settings: AttributesFormatString=%<FuncName>
  SrvResp : Outport  RequirementInfo="{'linktype_rmi_doors' '0000babb (/E-STEER Core/SubSystem Specifications/Application Functions/SF053A Handwheel Angle Vehicle Center Trim)' '#SF053A_28' 'true' 'REQ:  SF053A_28' '' } %GIDa_251bd858_14f9_4e1f_8195_733b734e112a"
  HwAgTrimPrfmd : Outport  RequirementInfo="{'linktype_rmi_doors' '0000babb (/E-STEER Core/SubSystem Specifications/Application Functions/SF053A Handwheel Angle Vehicle Center Trim)' '#SF053A_88' 'true' 'REQ:  SF053A_88' '' ; 'linktype_rmi_doors' '0000babb (/E-STEER Core/SubSystem Specifications/Application Functions/SF053A Handwheel Angle Vehicle Center Trim)' '#SF053A_91' 'true' 'REQ:  SF053A_91' '' } %GIDa_3a3571d3_5de0_4370_9484_523bb7c56762"  Port=2
  wires:
  Constant/1 -> SrvResp/1
  HwAg/1 -> HwAgTrimVal_Write/1
  Constant5/1 -> Set Ram Block Status/1
  Constant6/1 -> HwAgTrimPrfmd/1, HwAgTrimVal_Write/2

== system SF053A_HwAgVehCentrTrim/HwAgVehCentrTrim/UpdHwAgTrimVal/VehSpdThdExcdd ==
  Action Port : ActionPort  ActionType=then
  Constant : Constant  Value=VEHSPDTHDEXCDD_CNT_U08
  CopyRight2 : Subsystem  Description=|  mask(Copyright Information){none=on}
      | Copyright info block.                                               
      |                                                                     
      | Place copyright information at the top of every subsystem in design.
      mask prompts: none "No parameters"
      mask help: Place copyright information at the top of every subsystem in design.
      mask Display:
      | NxtrConf = 'Nexteer Confidential';
      | 
      | sys = bdroot; %handle for the current model ("system")
      | first = get_param(sys,'Created');
      | if(isempty(first))
      |     first = datestr(now,'yyyy');
      | else
      |     first = first(end-3:end);  %year is last four digits
      | end
      | 
      | last = get_param(sys,'LastModifiedDate');
      | if isempty(last)
      |     last = datestr(now,'yyyy');
      | else
      |     last = last(end-3:end);
      | end
      | 
      | if strcmp(first,last)
      |     fprintf('%s -- Copyright %s Nexteer',NxtrConf,first)
      | else
      |     fprintf('%s -- %s%s- %s Nexteer',NxtrConf,char(169),first,last)
      | end
  SrvResp : Outport
  wires:
  Constant/1 -> SrvResp/1

== system SF053A_HwAgVehCentrTrim/HwAgVehCentrTrim/ClrHwAgTrimVal/SetNtcSts/CopyRight2 ==

== system SF053A_HwAgVehCentrTrim/HwAgVehCentrTrim/HwAgVehCentrTrimInit1/SetNtcSts/CopyRight2 ==

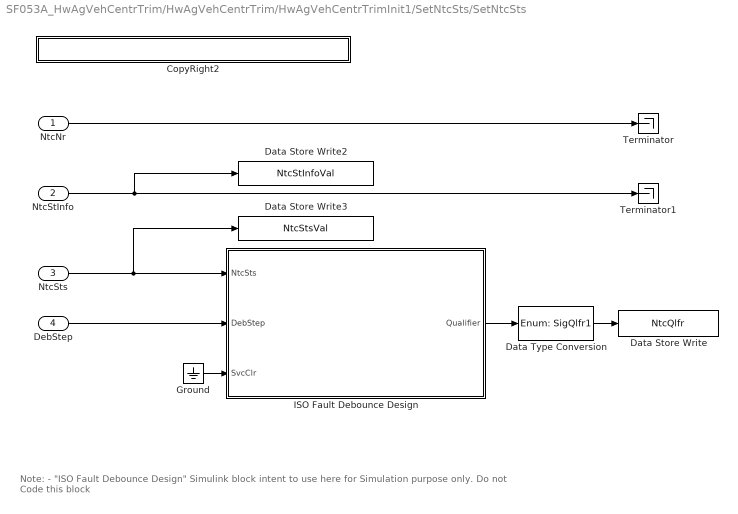
== system SF053A_HwAgVehCentrTrim/HwAgVehCentrTrim/HwAgVehCentrTrimInit1/SetNtcSts/SetNtcSts ==
  note: Note:
      |
      | - "ISO Fault Debounce Design" Simulink block intent to use here for Simulation purpose only. Do not Code this block
  NtcNr : Inport
  NtcStInfo : Inport  Port=2
  NtcSts : Inport  Port=3
  DebStep : Inport  Port=4
  CopyRight2 : Subsystem  Description=|  mask(Copyright Information){none=on}
      | Copyright info block.                                               
      |                                                                     
      | Place copyright information at the top of every subsystem in design.
      mask prompts: none "No parameters"
      mask help: Place copyright information at the top of every subsystem in design.
      mask Display:
      | NxtrConf = 'Nexteer Confidential';
      | 
      | sys = bdroot; %handle for the current model ("system")
      | first = get_param(sys,'Created');
      | first = first(end-3:end);  %year is last four digits
      | 
      | last = get_param(sys,'LastModifiedDate');
      | if isempty(last)
      |     last = datestr(now,'yyyy');
      | else
      |     last = last(end-3:end);
      | end
      | 
      | if strcmp(first,last)
      |     fprintf('%s -- Copyright %s Nexteer',NxtrConf,first)
      | else
      |     fprintf('%s -- %s%s- %s Nexteer',NxtrConf,char(169),first,last)
      | end
  Data Store Write : DataStoreWrite  DataStoreName=NtcQlfr
  Data Store Write2 : DataStoreWrite  DataStoreName=NtcStInfoVal
  Data Store Write3 : DataStoreWrite  DataStoreName=NtcStsVal
  Data Type Conversion : DataTypeConversion  OutDataTypeStr=Enum: SigQlfr1
  Ground : Ground
  ISO Fault Debounce Design : Stateflow chart  TreatAsAtomicUnit=on
      settings: AttributesFormatString=|
      | Simulation Purpose Only.
      | Do Not Code this block
      | Diagnostic Manager Owns this requirement
  Terminator : Terminator
  Terminator1 : Terminator
  wires:
  NtcStInfo/1 -> Data Store Write2/1, Terminator1/1
  NtcNr/1 -> Terminator/1
  NtcSts/1 -> Data Store Write3/1, ISO Fault Debounce Design/1(NtcSts)
  DebStep/1 -> ISO Fault Debounce Design/2(DebStep)
  ISO Fault Debounce Design/1(Qualifier) -> Data Type Conversion/1
  Ground/1 -> ISO Fault Debounce Design/3(SvcClr)
  Data Type Conversion/1 -> Data Store Write/1

== system SF053A_HwAgVehCentrTrim/HwAgVehCentrTrim/HwAgVehCentrTrimPer1/SetNtcSts/CopyRight2 ==
